simulink model "TestHeightController"  (R2017b)
settings: Solver=VariableStepAuto  StartTime=0.0  StopTime=10.0  RelTol=1e-3
undefined symbols (not defined in the file): Initial, Uav
libraries: QuaternionLibrary x5, simulink x1
settings Model: Creator=jban039  LastModifiedBy=jban039

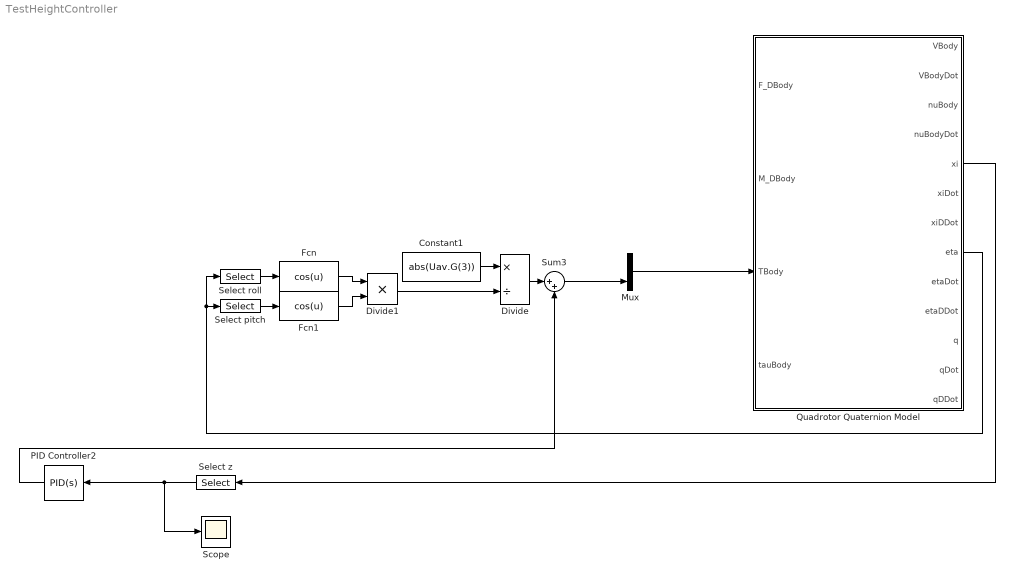
== system TestHeightController ==
  Constant1 : Constant  Value=abs(Uav.G(3))
  Divide : Product  Inputs=*/
  Divide1 : Product  Inputs=**
  Fcn : Fcn  Expr=cos(u)
  Fcn1 : Fcn  Expr=cos(u)
  Mux : Mux  Inputs=3
  PID Controller2 : simulink/Continuous/PID Controller  Controller=PID  TimeDomain=Continuous-time  SampleTime=-1  IntegratorMethod=Forward Euler  FilterMethod=Forward Euler  Form=Parallel  UseFilter=on  ControllerParametersSource=internal  P=-22.065410118279  I=-10.2297340963903  D=-11.7817329577601  N=104.897155810233  InitialConditionSource=internal  InitialConditionForIntegrator=0  InitialConditionForFilter=0  ExternalReset=none  LimitOutput=off  UpperSaturationLimit=inf  LowerSaturationLimit=-inf  LinearizeAsGain=on  AntiWindupMode=none  Kb=1  TrackingMode=off  Kt=1  PParamMin=[]  PParamMax=[]  IParamMin=[]  IParamMax=[]  DParamMin=[]  DParamMax=[]  NParamMin=[]  NParamMax=[]  KbParamMin=[]  KbParamMax=[]  KtParamMin=[]  KtParamMax=[]  POutMin=[]  POutMax=[]  IOutMin=[]  IOutMax=[]  DOutMin=[]  DOutMax=[]  NOutMin=[]  NOutMax=[]  KbOutMin=[]  KbOutMax=[]  KtOutMin=[]  KtOutMax=[]  IntegratorOutMin=[]  IntegratorOutMax=[]  FilterOutMin=[]  FilterOutMax=[]  SumOutMin=[]  SumOutMax=[]  SumI1OutMin=[]  SumI1OutMax=[]  SumI2OutMin=[]  SumI2OutMax=[]  SumI3OutMin=[]  SumI3OutMax=[]  SumDOutMin=[]  SumDOutMax=[]  SaturationOutMin=[]  SaturationOutMax=[]  IntegratorContinuousStateAttributes=''  IntegratorStateMustResolveToSignalObject=off  IntegratorRTWStateStorageClass=Auto  FilterContinuousStateAttributes=''  FilterStateMustResolveToSignalObject=off  FilterRTWStateStorageClass=Auto  DifferentiatorICPrevScaledInput=0  DifferentiatorOutMin=[]  DifferentiatorOutMax=[]  InitialConditionSetting=State (most efficient)  FilterDiffOutCoefMin=[]  FilterDiffOutCoefMax=[]  SumDenOutMin=[]  SumDenOutMax=[]  SumNumOutMin=[]  SumNumOutMax=[]  ReciprocalOutMin=[]  ReciprocalOutMax=[]  DivideOutMin=[]  DivideOutMax=[]  TunerSelectOption=Transfer Function Based (PID Tuner App)
  Quadrotor Quaternion Model : Subsystem
  Scope : Scope
  Select pitch : Selector  InputPortWidth=3  IndexOptions=Index vector (dialog)  Indices=2  OutputSizes=1
  Select roll : Selector  InputPortWidth=3  IndexOptions=Index vector (dialog)  Indices=1  OutputSizes=1
  Select z : Selector  InputPortWidth=3  IndexOptions=Index vector (dialog)  Indices=3  OutputSizes=1
  Sum3 : Sum  Inputs=|++
  wires:
  PID Controller2/1 -> Sum3/2
  Divide1/1 -> Divide/2
  Fcn1/1 -> Divide1/2
  Fcn/1 -> Divide1/1
  Select pitch/1 -> Fcn1/1
  Select roll/1 -> Fcn/1
  Quadrotor Quaternion Model/8(eta) -> Select pitch/1, Select roll/1
  Constant1/1 -> Divide/1
  Divide/1 -> Sum3/1
  Sum3/1 -> Mux/3
  Mux/1 -> Quadrotor Quaternion Model/3(TBody)
  Quadrotor Quaternion Model/5(xi) -> Select z/1
  Select z/1 -> Scope/1, PID Controller2/1

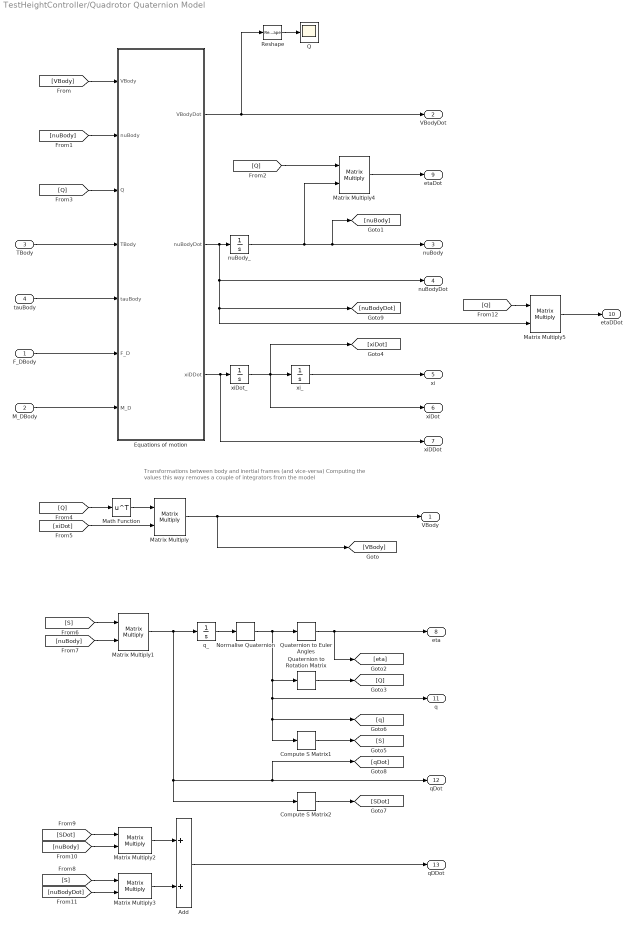
== system TestHeightController/Quadrotor Quaternion Model ==
  note: Transformations between body and inertial frames (and vice-versa)
      | Computing the values this way removes a couple of integrators from the model
  F_DBody : Inport  Unit=N
  M_DBody : Inport  Port=2  Unit=N*m
  TBody : Inport  Port=3  Unit=N
  tauBody : Inport  Port=4  Unit=N*m
  Add : Sum
  Compute S Matrix1 : QuaternionLibrary/Compute S Matrix
  Compute S Matrix2 : QuaternionLibrary/Compute S Matrix
  Equations of motion : MATLAB Function  TreatAsAtomicUnit=on
  Math Function : Math  Operator=transpose  SaturateOnIntegerOverflow=on
  Matrix Multiply{,1..5} (6 alike) : Product  Multiplication=Matrix(*)
  Normalise Quaternion : QuaternionLibrary/Normalise Quaternion
  Q : Scope
  Quaternion to Euler Angles : QuaternionLibrary/Quaternion to Euler Angles
  Quaternion to Rotation Matrix : QuaternionLibrary/Quaternion to Rotation Matrix
  Reshape : Reshape  OutputDimensionality=Column vector (2-D)
  nuBody_ : Integrator  InitialCondition=Initial.NU_BODY
  q_ : Integrator  InitialCondition=Initial.Q
  xiDot_ : Integrator  InitialCondition=Initial.XI_DOT
  xi_ : Integrator  InitialCondition=[0;0;0.01]
  VBody : Outport  Unit=m/s
  VBodyDot : Outport  Port=2  Unit=m/s^2
  nuBody : Outport  Port=3  Unit=rad/s
  nuBodyDot : Outport  Port=4  Unit=rad/s^2
  xi : Outport  Port=5  Unit=m
  xiDot : Outport  Port=6  Unit=m/s
  xiDDot : Outport  Port=7  Unit=m/s^2
  eta : Outport  Port=8  Unit=rad
  etaDot : Outport  Port=9  Unit=rad/s
  etaDDot : Outport  Port=10  Unit=rad/s^2
  q : Outport  Port=11
  qDot : Outport  Port=12
  qDDot : Outport  Port=13
  wires:
  xiDot_/1 -> xiDot/1, [xiDot], xi_/1
  Reshape/1 -> Q/1
  Matrix Multiply5/1 -> etaDDot/1
  [Q] -> Matrix Multiply5/1
  Add/1 -> qDDot/1
  [Q] -> Matrix Multiply4/1
  Compute S Matrix1/1 -> [S]
  Normalise Quaternion/1 -> Quaternion to Rotation Matrix/1, [q], Compute S Matrix1/1, q/1, Quaternion to Euler Angles/1
  Matrix Multiply3/1 -> Add/2
  Matrix Multiply2/1 -> Add/1
  [nuBodyDot] -> Matrix Multiply3/2
  [nuBody] -> Matrix Multiply2/2
  [SDot] -> Matrix Multiply2/1
  Matrix Multiply1/1 -> q_/1, Compute S Matrix2/1, [qDot], qDot/1
  [S] -> Matrix Multiply3/1
  Compute S Matrix2/1 -> [SDot]
  [nuBody] -> Matrix Multiply1/2
  [S] -> Matrix Multiply1/1
  Math Function/1 -> Matrix Multiply/1
  [xiDot] -> Matrix Multiply/2
  [Q] -> Math Function/1
  [Q] -> Equations of motion/3(Q)
  Quaternion to Rotation Matrix/1 -> [Q]
  Matrix Multiply4/1 -> etaDot/1
  Quaternion to Euler Angles/1 -> [eta], eta/1
  q_/1 -> Normalise Quaternion/1
  Equations of motion/2(nuBodyDot) -> [nuBodyDot], Matrix Multiply5/2, nuBodyDot/1, nuBody_/1
  nuBody_/1 -> nuBody/1, [nuBody], Matrix Multiply4/2
  M_DBody/1 -> Equations of motion/7(M_D)
  Matrix Multiply/1 -> [VBody], VBody/1
  F_DBody/1 -> Equations of motion/6(F_D)
  Equations of motion/3(xiDDot) -> xiDDot/1, xiDot_/1
  TBody/1 -> Equations of motion/4(TBody)
  tauBody/1 -> Equations of motion/5(tauBody)
  [VBody] -> Equations of motion/1(VBody)
  [nuBody] -> Equations of motion/2(nuBody)
  xi_/1 -> xi/1
  Equations of motion/1(VBodyDot) -> VBodyDot/1, Reshape/1

== matlab function TestHeightController/Quadrotor Quaternion Model/Equations of motion ==
  data: VBody input; VBodyDot output; nuBody input; Q input; TBody input size=3; tauBody input size=3; F_D input size=3; M_D input size=3; nuBodyDot output; Uav parameter; xiDDot output
function [VBodyDot, nuBodyDot, xiDDot] = QuadrotorQuaternionModel(...
    VBody, nuBody, Q, TBody, tauBody, F_D, M_D, Uav)
%#codegen

%% Rotation matrices

%% Moments and Forces
% Body frame accelerations
VBodyDot  = (1/Uav.M) * (Q'*Uav.G + TBody - cross(nuBody, Uav.M*VBody) - F_D);
nuBodyDot = Uav.I \ (tauBody - cross(nuBody, Uav.I*nuBody) - M_D);

% Inertial frame accelerations
xiDDot = (1/Uav.M)*(Uav.G + Q*(TBody - F_D));
% etaDDot = WInvertDot*nuBody + WInvert*nuBodyDot;

% Check centripetal force in inertial frame
% F_C = R*cross(nuBody,m*VBody);
end
